simulink model "PAlab4simulink"  (R2019a)
settings: Solver=VariableStepAuto  StartTime=0.0  StopTime=20  RelTol=1e-3
settings Model: Creator=ASUS_PEPE  LastModifiedBy=ASUS_PEPE

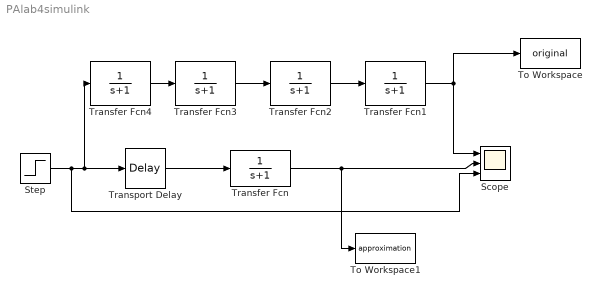
== system PAlab4simulink ==
  Scope : Scope  NumInputPorts=3
  Step : Step  Before=1  SampleTime=0
  To Workspace : ToWorkspace  VariableName=original  SaveFormat=Timeseries  SampleTime=-1
  To Workspace1 : ToWorkspace  VariableName=approximation  SaveFormat=Timeseries  SampleTime=-1
  Transfer Fcn{,1..4} (5 alike) : TransferFcn  Denominator=[1 1]
  Transport Delay : TransportDelay  DelayTime=11
  wires:
  Step/1 -> Scope/3, Transfer Fcn4/1, Transport Delay/1
  Transport Delay/1 -> Transfer Fcn/1
  Transfer Fcn/1 -> To Workspace1/1, Scope/2
  Transfer Fcn1/1 -> To Workspace/1, Scope/1
  Transfer Fcn4/1 -> Transfer Fcn3/1
  Transfer Fcn3/1 -> Transfer Fcn2/1
  Transfer Fcn2/1 -> Transfer Fcn1/1
